simulink model "test_identification"  (Simulink 6.5)
settings: Solver=ode45  StartTime=0.0  StopTime=L  RelTol=1e-6
undefined symbols (not defined in the file): K, Kd, L, M_ecart, N, Tau, Tc, Te, Vit
libraries: simulink_extras x1
settings Model: Creator=admin  LastModifiedBy=admin
settings DataIOCC: SignalLoggingName=sigsOut
settings DebuggingCC: SolverPrmCheckMsg=none  MultiTaskDSMMsg=warning  MultiTaskCondExecSysMsg=none  StrictBusMsg=None
settings HardwareCC: TargetUnknown=on
settings RTWCC: IncludeERTFirstTime=on

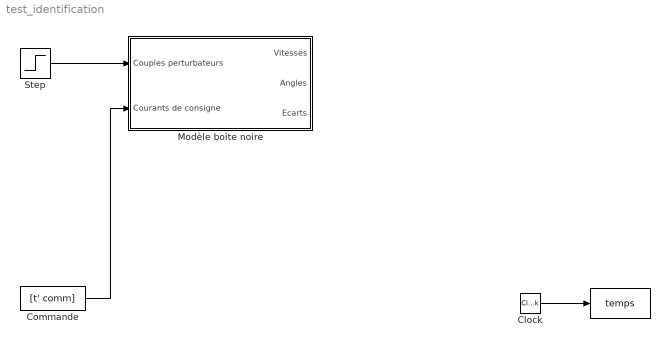
== system test_identification ==
  " " : ToWorkspace  VariableName=temps  SampleTime=-1  SaveFormat=Array
  Clock : DigitalClock  SampleTime=Te
  Commande : FromWorkspace  VariableName=[t' comm]  SampleTime=Tc
  Modèle boîte noire : Subsystem
  Step : Step  Time=L*0.1  Before=zeros(N,1)  After=zeros(N,1)
  wires:
  Step/1 -> Modèle boîte noire/1(Couples perturbateurs)
  Clock/1 -> " "/1
  Commande/1 -> Modèle boîte noire/2(Courants de consigne)

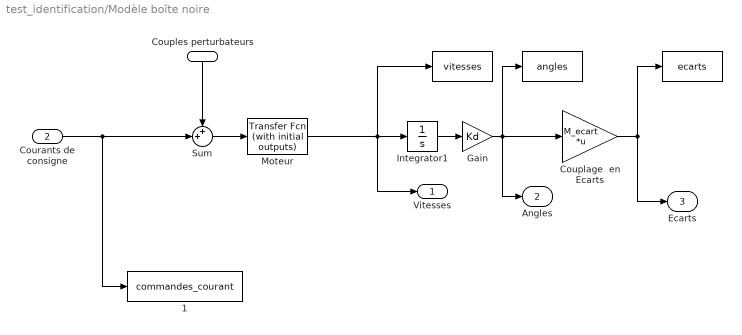
== system test_identification/Modèle boîte noire ==
  Couples perturbateurs : Inport  Orientation=down
  Courants de consigne : Inport  Port=2
  " " : ToWorkspace  VariableName=vitesses  SampleTime=Te  SaveFormat=Array
  "  " : ToWorkspace  VariableName=angles  SampleTime=Te  SaveFormat=Array
  "   " : ToWorkspace  VariableName=ecarts  SampleTime=Te  SaveFormat=Array
  "   1" : ToWorkspace  VariableName=commandes_courant  SampleTime=-1  SaveFormat=Array
  Couplage  en Ecarts : Gain  Gain=M_ecart  Multiplication=Matrix(K*u)  SaturateOnIntegerOverflow=on
  Gain : Gain  Gain=Kd
  Integrator1 : Integrator  InitialCondition=927/Kd
  Moteur : simulink_extras/Additional Linear/Transfer Fcn (with initial outputs)  SystemSampleTime=-1  N=[K]  D="[Tau  1]"  Y0=Vit(1)  U0=Vit(1)
  Sum : Sum  Inputs=++|  SaturateOnIntegerOverflow=on
  Vitesses : Outport
  Angles : Outport  Port=2
  Ecarts : Outport  Port=3
  wires:
  Couplage  en Ecarts/1 -> Ecarts/1, "   "/1
  Courants de consigne/1 -> "   1"/1, Sum/2
  Couples perturbateurs/1 -> Sum/1
  Integrator1/1 -> Gain/1
  Sum/1 -> Moteur/1
  Moteur/1 -> Integrator1/1, " "/1, Vitesses/1
  Gain/1 -> Couplage  en Ecarts/1, Angles/1, "  "/1
